simulink model "linmodel_eq1_discr_PID"  (R2019a)
settings: Solver=VariableStepAuto  StartTime=0.0  StopTime=30  RelTol=1e-3
InitFcn:
  | lin_discr_model
values from neighbouring files (symbols this model uses):
  A_eq1_d = sysd1.A    [lin_discr_model_PID.m]
  B_eq1_d = sysd1.B    [lin_discr_model_PID.m]
  C_eq1_d = sysd1.C    [lin_discr_model_PID.m]
  Ts = 0.01    [lin_discr_model_PID.m]
undefined symbols (not defined in the file or in its folder): L
libraries: simulink x1
settings Model: Creator=jessi  LastModifiedBy=jessi

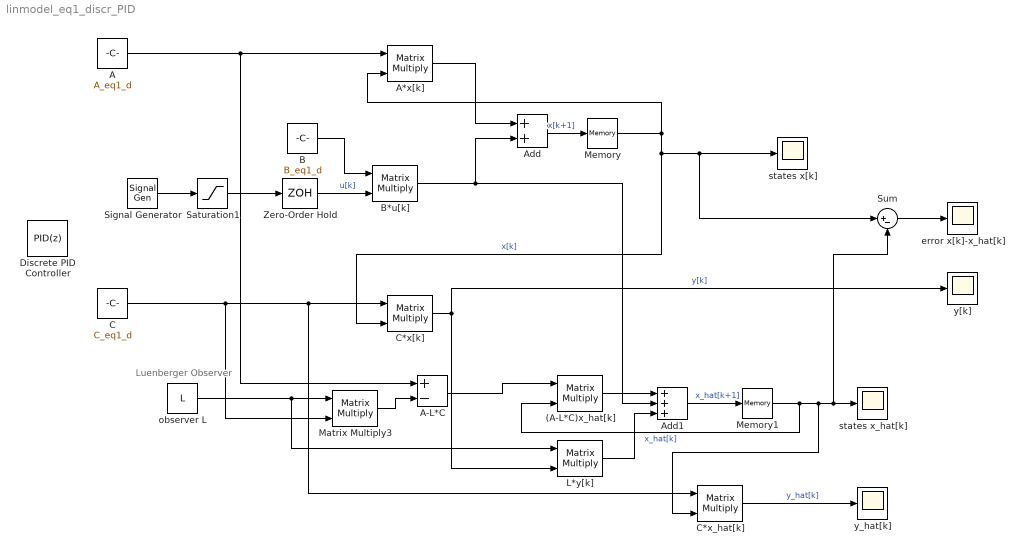
== system linmodel_eq1_discr_PID ==
  note: Luenberger Observer
  (A-L*C)x_hat[k] : Product  Multiplication=Matrix(*)
  A : Constant  Value=A_eq1_d  SampleTime=Ts
  A*x[k] : Product  Multiplication=Matrix(*)
  A-L*C : Sum  Inputs=+-
  Add : Sum
  Add1 : Sum  Inputs=+++
  B : Constant  Value=B_eq1_d  SampleTime=Ts
  B*u[k] : Product  Multiplication=Matrix(*)
  C : Constant  Value=C_eq1_d  SampleTime=Ts
  C*x[k] : Product  Multiplication=Matrix(*)
  C*x_hat[k] : Product  Multiplication=Matrix(*)
  Discrete PID Controller : simulink/Continuous/PID Controller  Controller=PID  Form=Parallel  TimeDomain=Discrete-time  SampleTime=Ts  IntegratorMethod=Forward Euler  FilterMethod=Forward Euler  ControllerParametersSource=internal  P=1  I=1  D=0  UseFilter=on  N=100  TunerSelectOption=Transfer Function Based (PID Tuner App)  InitialConditionSource=internal  InitialConditionForIntegrator=0  InitialConditionForFilter=0  DifferentiatorICPrevScaledInput=0  ExternalReset=none  TrackingMode=off  Kt=1  LimitOutput=off  UpperSaturationLimit=inf  LowerSaturationLimit=-inf  LinearizeAsGain=off  AntiWindupMode=none  Kb=1  POutMin=[]  POutMax=[]  IOutMin=[]  IOutMax=[]  DOutMin=[]  DOutMax=[]  NOutMin=[]  NOutMax=[]  SumOutMin=[]  SumOutMax=[]  SaturationOutMin=[]  SaturationOutMax=[]  PParamMin=[]  PParamMax=[]  IParamMin=[]  IParamMax=[]  DParamMin=[]  DParamMax=[]  NParamMin=[]  NParamMax=[]  KbParamMin=[]  KbParamMax=[]  KtParamMin=[]  KtParamMax=[]  KbOutMin=[]  KbOutMax=[]  KtOutMin=[]  KtOutMax=[]  IntegratorOutMin=[]  IntegratorOutMax=[]  FilterOutMin=[]  FilterOutMax=[]  SumI1OutMin=[]  SumI1OutMax=[]  SumI2OutMin=[]  SumI2OutMax=[]  SumI3OutMin=[]  SumI3OutMax=[]  SumI4OutMin=[]  SumI4OutMax=[]  SumDOutMin=[]  SumDOutMax=[]  DifferentiatorOutMin=[]  DifferentiatorOutMax=[]  FilterDiffOutCoefMin=[]  FilterDiffOutCoefMax=[]  ReciprocalOutMin=[]  ReciprocalOutMax=[]  SumDenOutMin=[]  SumDenOutMax=[]  SumNumOutMin=[]  SumNumOutMax=[]  DivideOutMin=[]  DivideOutMax=[]  IntegratorContinuousStateAttributes=''  IntegratorStateMustResolveToSignalObject=off  IntegratorRTWStateStorageClass=Auto  FilterContinuousStateAttributes=''  FilterStateMustResolveToSignalObject=off  FilterRTWStateStorageClass=Auto  ParallelPVariant=InternalParameters  IdealPVariant=Disabled  IVariant=InternalParameters  DVariant=InternalParameters  IntegratorVariant=Discrete  SatVariant=Disabled  AWVariant=Passthrough  PCopyVariant=Disabled  TRVariant=Disabled  FdbkBlocksVariant=Forward  IdealPFdbkVariant=Disabled  SatFdbkVariant=Disabled  DerivativeFilterVariant=ForwardEulerFilter  NVariant=InternalParameters  NCopyVariant=Disabled  FilterICVariant=InternalICsFilter  IntegratorICVariant=InternalICs  ExternalResetVariant=Disabled  TRSumVariant=Passthrough  SumFdbkVariant=Disabled  SumVariant=Sum_PID
  L*y[k] : Product  Multiplication=Matrix(*)
  Matrix Multiply3 : Product  Multiplication=Matrix(*)
  Memory : Memory  InitialCondition=[pi;0;0;0]
  Memory1 : Memory  InitialCondition=[pi;0;0;0]
  Saturation1 : Saturate  UpperLimit=1  LowerLimit=-1
  Signal Generator : SignalGenerator  WaveForm=square  Amplitude=-0.3
  Sum : Sum  Inputs=|+-
  Zero-Order Hold : ZeroOrderHold  SampleTime=Ts
  error x[k]-x_hat[k] : Scope
  observer L : Constant  Value=L  SampleTime=Ts
  states x[k] : Scope
  states x_hat[k] : Scope
  y[k] : Scope
  y_hat[k] : Scope
  wires:
  Signal Generator/1 -> Saturation1/1
  Zero-Order Hold/1 -> B*u[k]/2  "u[k]"
  B/1 -> B*u[k]/1
  A/1 -> A-L*C/1, A*x[k]/1
  A*x[k]/1 -> Add/1
  B*u[k]/1 -> Add1/2, Add/2
  Memory/1 -> A*x[k]/2, Sum/1, states x[k]/1, C*x[k]/2  "x[k]"
  C/1 -> Matrix Multiply3/2, C*x_hat[k]/1, C*x[k]/1
  C*x[k]/1 -> L*y[k]/2, y[k]/1  "y[k]"
  observer L/1 -> L*y[k]/1, Matrix Multiply3/1
  Matrix Multiply3/1 -> A-L*C/2
  A-L*C/1 -> (A-L*C)x_hat[k]/1
  (A-L*C)x_hat[k]/1 -> Add1/1
  L*y[k]/1 -> Add1/3
  Add1/1 -> Memory1/1  "x_hat[k+1]"
  Memory1/1 -> C*x_hat[k]/2, Sum/2, states x_hat[k]/1, (A-L*C)x_hat[k]/2  "x_hat[k]"
  C*x_hat[k]/1 -> y_hat[k]/1  "y_hat[k]"
  Saturation1/1 -> Zero-Order Hold/1
  Add/1 -> Memory/1  "x[k+1]"
  Sum/1 -> error x[k]-x_hat[k]/1
